simulink model "test_VisionModel_v1"  (Simulink 7.6)
settings: Solver=FixedStepDiscrete  StartTime=0.0  StopTime=0  RelTol=1e-3
values from neighbouring files (symbols this model uses):
  Scale_Down_B = 1    [VisionConstants.m]
  Scale_Down_G = 1    [VisionConstants.m]
  Scale_Down_H = 1    [VisionConstants.m]
  Scale_Down_R = 1    [VisionConstants.m]
  Scale_Down_S = 1    [VisionConstants.m]
  Scale_Down_V = 5    [VisionConstants.m]
  Scale_Forward_B = 0    [VisionConstants.m]
  Scale_Forward_G = 1    [VisionConstants.m]
  Scale_Forward_H = 1    [VisionConstants.m]
  Scale_Forward_R = 0    [VisionConstants.m]
  Scale_Forward_S = 1    [VisionConstants.m]
  Scale_Forward_V = 5    [VisionConstants.m]
undefined symbols (not defined in the file or in its folder): gray, Rec, SDTV
libraries: vipconversions x7, vipsnks x6, vipsrcs x2, viptextngfix x1
settings Model: Creator=Thing 1  LastModifiedBy=auvt
settings OptimizationCC: InlineParams=on  OptimizeModelRefInitCode=on
settings RTWCC: SystemTargetFile=ert.tlc  GenCodeOnly=on  TemplateMakefile=ert_default_tmf  Description=Real-Time Workshop Embedded Coder  GenerateReport=on  ProcessScript=ert_make_rtw_hook  IncludeHyperlinkInReport=on  LaunchReport=on  TargetLang=C++
settings CodeAppCC: IgnoreCustomStorageClasses=off
settings ERTTargetCC: MultiwordLength=2048  GenerateSampleERTMain=on  IncludeMdlTerminateFcn=off  ERTCustomFileTemplate=example_file_process.tlc  ConvertIfToSwitch=off

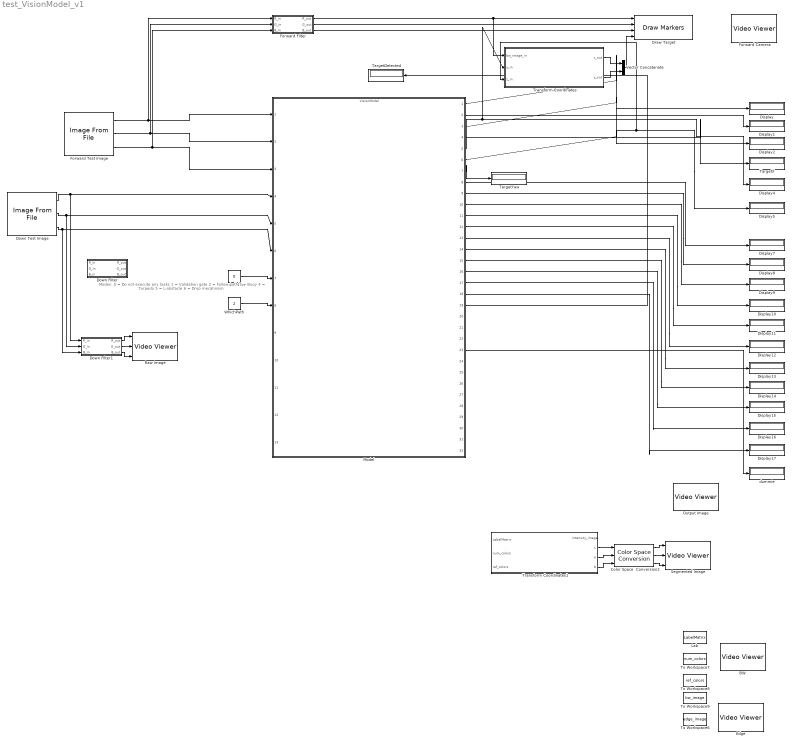
== system test_VisionModel_v1 ==
  note: Modes:
      | 0 = Do not execute any tasks
      | 1 = Validation gate
      | 2 = Follow path
      | 3 = Buoy
      | 4 = Torpedo
      | 5 = L-obstacle
      | 6 = Drop mecahnism
  BW : vipsnks/Video Viewer  DialogControllerArgs=DataTag1  inputType=Obsolete7b  imagePorts=One multidimensional signal  useColorMap=off  colormapValue=gray(256)  specRange=off  minInputVal=0  maxInputVal=255  FigPos=[569 648 462 512]  AxisZoom=on  trueSizedOnce=off  OpenAtMdlStart=on
  Color Space  Conversion2 : vipconversions/Color Space  Conversion  conversion=Obsolete  conversionActive=L*a*b* to sR'G'B'  wp_str=D50  rec=Rec. 601 (SDTV)  sys=1125/60/2:1  imagePorts=Separate color signals
  Display{,1..2,4..5,7..17} (16 alike) : Display
  Down Filter : Subsystem
  Down Filter1 : Subsystem
  Down Test Image : vipsrcs/Image From File  Tag=vipblks_nd  DialogController=vipDDGCreate  DialogControllerArgs=DataTag2  SystemSampleTime=-1  FileName=/home/auvt/auvc/src/vision/Test_Images/path10.bmp  imagePorts=Separate color signals  Ts=-1  ImageDataType=double  Signed=on  WordLength=16  sdImageDataType=uint(8)  FractionLengthMode=User-defined  FractionLength=15  OutPortLabels=R|G|B
  Draw Target : viptextngfix/Draw Markers  DialogController=vipDDGCreate  DialogControllerArgs=DataTag3  shape=X-mark  size=7  fill=off  fillClrSource=Specify via dialog  display=User-specified value  intensity=200  color=[0 0 0]  opacity=0.6  viewport=Entire image  antialiasing=off  inType=Obsolete  imagePorts=Separate color signals  prodOutputMode=Binary point scaling  prodOutputWordLength=32  prodOutputFracLength=14  memoryMode=Specify word length  memoryWordLength=16  memoryFracLength=15  roundingMode=Floor  overflowMode=off
  Edge : vipsnks/Video Viewer  DialogControllerArgs=DataTag5  inputType=Obsolete7b  imagePorts=One multidimensional signal  useColorMap=off  colormapValue=gray(256)  specRange=off  minInputVal=0  maxInputVal=255  FigPos=[58 764 334 594]  AxisZoom=on  trueSizedOnce=off  OpenAtMdlStart=on
  Forward Camera : vipsnks/Video Viewer  DialogControllerArgs=DataTag7  inputType=Obsolete7b  imagePorts=Separate color signals  useColorMap=off  colormapValue=gray(256)  specRange=off  minInputVal=0  maxInputVal=255  FigPos=[1018 735 364 553]  AxisZoom=on  trueSizedOnce=off  OpenAtMdlStart=on
  Forward Filter : Subsystem
  Forward Test Image : vipsrcs/Image From File  Tag=vipblks_nd  DialogController=vipDDGCreate  DialogControllerArgs=DataTag8  SystemSampleTime=-1  FileName=/home/auvt/auvc/src/vision/Test_Images/gate13.bmp  imagePorts=Separate color signals  Ts=-1  ImageDataType=double  Signed=on  WordLength=16  sdImageDataType=uint(8)  FractionLengthMode=User-defined  FractionLength=15  OutPortLabels=R|G|B
  Lab : ToWorkspace  VariableName=LabelMatrix  SampleTime=-1  SaveFormat=Array
  ModeSelect : Constant  Value=0  SampleTime=-1
  Model : ModelReference  ModelNameDialog=VisionModel  SimulationMode=Accelerator  ModelReferenceVersion=1.469  CopyOfModelName=VisionModel
  Output Image : vipsnks/Video Viewer  DialogControllerArgs=DataTag10  inputType=Obsolete7b  imagePorts=Separate color signals  useColorMap=off  colormapValue=gray(256)  specRange=off  minInputVal=0  maxInputVal=255  FigPos=[957 861 423 448]  AxisZoom=on  trueSizedOnce=off  OpenAtMdlStart=on
  Raw Image : vipsnks/Video Viewer  DialogControllerArgs=DataTag12  inputType=Obsolete7b  imagePorts=Separate color signals  useColorMap=off  colormapValue=gray(256)  specRange=off  minInputVal=0  maxInputVal=255  FigPos=[110 703 515 461]  AxisZoom=on  trueSizedOnce=off  OpenAtMdlStart=on
  Segmented Image : vipsnks/Video Viewer  DialogControllerArgs=DataTag14  inputType=Obsolete7b  imagePorts=Separate color signals  useColorMap=off  colormapValue=gray(256)  specRange=off  minInputVal=0  maxInputVal=255  FigPos=[955 778 266 280]  AxisZoom=on  trueSizedOnce=off  OpenAtMdlStart=on
  TargetDetected : Display
  TargetX : Display
  TargetYaw : Display
  To Workspace6 : ToWorkspace  VariableName=edge_image  SampleTime=-1  SaveFormat=Array
  To Workspace7 : ToWorkspace  VariableName=num_colors  SampleTime=-1  SaveFormat=Array
  To Workspace8 : ToWorkspace  VariableName=ref_colors  SampleTime=-1  SaveFormat=Array
  To Workspace9 : ToWorkspace  VariableName=bw_image  SampleTime=-1  SaveFormat=Array
  Transform Coordinates : Stateflow chart  TreatAsAtomicUnit=on  SystemSampleTime=[1/30 0]
  Transform Coordinates1 : Stateflow chart  TreatAsAtomicUnit=on  SystemSampleTime=[1/30 0]
  Vector Concatenate : Concatenate  Mode=Multidimensional array
  WhichPath : Constant  Value=2  SampleTime=-1
  dummie : Display
  wires:
  Down Test Image/1 -> Model/4, Down Filter1/1(R_in)
  Down Test Image/2 -> Model/5, Down Filter1/2(G_in)
  Down Test Image/3 -> Model/6, Down Filter1/3(B_in)
  Model/1 -> Display/1
  Model/2 -> Display1/1
  Model/3 -> Display2/1
  Model/4 -> TargetX/1
  Model/8 -> Display7/1
  Model/9 -> Display8/1
  Model/10 -> Display9/1
  Model/11 -> Display10/1
  Model/12 -> Display11/1
  Model/13 -> Display12/1
  Model/14 -> Display13/1
  Model/15 -> Display14/1
  Model/16 -> Display15/1
  Model/17 -> Display16/1
  Model/18 -> Display17/1
  Transform Coordinates/1(x_out) -> Vector Concatenate/1
  Transform Coordinates/2(y_out) -> Vector Concatenate/2
  Vector Concatenate/1 -> Draw Target/4
  Forward Filter/1(R_out) -> Draw Target/1, Transform Coordinates/1(bw_image_in)
  Forward Filter/2(G_out) -> Draw Target/2
  Forward Filter/3(B_out) -> Draw Target/3
  Model/19 -> TargetDetected/1
  Model/23 -> dummie/1
  Model/5 -> Display4/1, Transform Coordinates/2(y_in)
  Model/6 -> Display5/1, Transform Coordinates/3(z_in)
  Forward Test Image/1 -> Model/1, Forward Filter/1(R_in)
  Forward Test Image/2 -> Model/2, Forward Filter/2(G_in)
  Forward Test Image/3 -> Model/3, Forward Filter/3(B_in)
  ModeSelect/1 -> Model/7
  WhichPath/1 -> Model/8
  Color Space  Conversion2/1 -> Segmented Image/1
  Color Space  Conversion2/2 -> Segmented Image/2
  Color Space  Conversion2/3 -> Segmented Image/3
  Transform Coordinates1/2(L) -> Color Space  Conversion2/1
  Transform Coordinates1/3(a) -> Color Space  Conversion2/2
  Transform Coordinates1/4(b) -> Color Space  Conversion2/3
  Model/7 -> TargetYaw/1
  Down Filter1/2(G_out) -> Raw Image/2
  Down Filter1/1(R_out) -> Raw Image/1
  Down Filter1/3(B_out) -> Raw Image/3

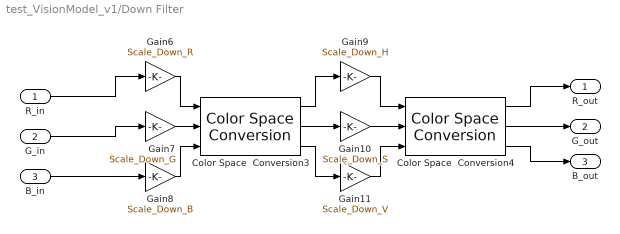
== system test_VisionModel_v1/Down Filter ==
  R_in : Inport  PortDimensions=Down_Camera_Dimensions
  G_in : Inport  Port=2  PortDimensions=Down_Camera_Dimensions
  B_in : Inport  Port=3  PortDimensions=Down_Camera_Dimensions
  Color Space  Conversion3 : vipconversions/Color Space  Conversion  conversion=Obsolete  conversionActive=R'G'B' to HSV  wp_str=D50  rec=Rec. 601 (SDTV)  sys=1125/60/2:1  imagePorts=Separate color signals
  Color Space  Conversion4 : vipconversions/Color Space  Conversion  conversion=Obsolete  conversionActive=HSV to R'G'B'  wp_str=D50  rec=Rec. 601 (SDTV)  sys=1125/60/2:1  imagePorts=Separate color signals
  Gain10 : Gain  Gain=Scale_Down_S
  Gain11 : Gain  Gain=Scale_Down_V
  Gain6 : Gain  Gain=Scale_Down_R
  Gain7 : Gain  Gain=Scale_Down_G
  Gain8 : Gain  Gain=Scale_Down_B
  Gain9 : Gain  Gain=Scale_Down_H
  R_out : Outport  OutDataTypeStr=double
  G_out : Outport  Port=2  OutDataTypeStr=double
  B_out : Outport  Port=3  OutDataTypeStr=double
  wires:
  Gain6/1 -> Color Space  Conversion3/1
  Gain7/1 -> Color Space  Conversion3/2
  Gain8/1 -> Color Space  Conversion3/3
  Color Space  Conversion3/1 -> Gain9/1
  Color Space  Conversion3/2 -> Gain10/1
  Color Space  Conversion3/3 -> Gain11/1
  Gain9/1 -> Color Space  Conversion4/1
  Gain10/1 -> Color Space  Conversion4/2
  Gain11/1 -> Color Space  Conversion4/3
  R_in/1 -> Gain6/1
  G_in/1 -> Gain7/1
  B_in/1 -> Gain8/1
  Color Space  Conversion4/1 -> R_out/1
  Color Space  Conversion4/2 -> G_out/1
  Color Space  Conversion4/3 -> B_out/1

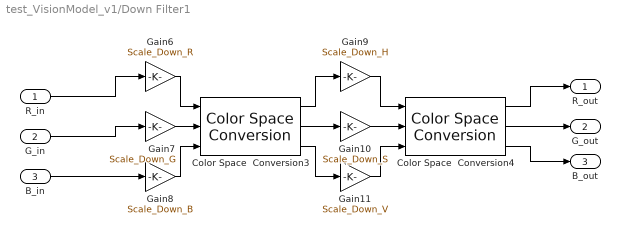
== system test_VisionModel_v1/Down Filter1 ==
  R_in : Inport  PortDimensions=Down_Camera_Dimensions
  G_in : Inport  Port=2  PortDimensions=Down_Camera_Dimensions
  B_in : Inport  Port=3  PortDimensions=Down_Camera_Dimensions
  Color Space  Conversion3 : vipconversions/Color Space  Conversion  conversion=Obsolete  conversionActive=R'G'B' to HSV  wp_str=D50  rec=Rec. 601 (SDTV)  sys=1125/60/2:1  imagePorts=Separate color signals
  Color Space  Conversion4 : vipconversions/Color Space  Conversion  conversion=Obsolete  conversionActive=HSV to R'G'B'  wp_str=D50  rec=Rec. 601 (SDTV)  sys=1125/60/2:1  imagePorts=Separate color signals
  Gain10 : Gain  Gain=Scale_Down_S
  Gain11 : Gain  Gain=Scale_Down_V
  Gain6 : Gain  Gain=Scale_Down_R
  Gain7 : Gain  Gain=Scale_Down_G
  Gain8 : Gain  Gain=Scale_Down_B
  Gain9 : Gain  Gain=Scale_Down_H
  R_out : Outport  OutDataTypeStr=double
  G_out : Outport  Port=2  OutDataTypeStr=double
  B_out : Outport  Port=3  OutDataTypeStr=double
  wires:
  Gain6/1 -> Color Space  Conversion3/1
  Gain7/1 -> Color Space  Conversion3/2
  Gain8/1 -> Color Space  Conversion3/3
  Color Space  Conversion3/1 -> Gain9/1
  Color Space  Conversion3/2 -> Gain10/1
  Color Space  Conversion3/3 -> Gain11/1
  Gain9/1 -> Color Space  Conversion4/1
  Gain10/1 -> Color Space  Conversion4/2
  Gain11/1 -> Color Space  Conversion4/3
  R_in/1 -> Gain6/1
  G_in/1 -> Gain7/1
  B_in/1 -> Gain8/1
  Color Space  Conversion4/1 -> R_out/1
  Color Space  Conversion4/2 -> G_out/1
  Color Space  Conversion4/3 -> B_out/1

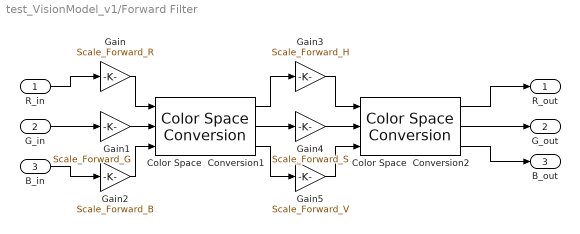
== system test_VisionModel_v1/Forward Filter ==
  R_in : Inport  PortDimensions=Forward_Camera_Dimensions
  G_in : Inport  Port=2  PortDimensions=Forward_Camera_Dimensions
  B_in : Inport  Port=3  PortDimensions=Forward_Camera_Dimensions
  Color Space  Conversion1 : vipconversions/Color Space  Conversion  conversion=Obsolete  conversionActive=R'G'B' to HSV  wp_str=D50  rec=Rec. 601 (SDTV)  sys=1125/60/2:1  imagePorts=Separate color signals
  Color Space  Conversion2 : vipconversions/Color Space  Conversion  conversion=Obsolete  conversionActive=HSV to R'G'B'  wp_str=D50  rec=Rec. 601 (SDTV)  sys=1125/60/2:1  imagePorts=Separate color signals
  Gain : Gain  Gain=Scale_Forward_R
  Gain1 : Gain  Gain=Scale_Forward_G
  Gain2 : Gain  Gain=Scale_Forward_B
  Gain3 : Gain  Gain=Scale_Forward_H
  Gain4 : Gain  Gain=Scale_Forward_S
  Gain5 : Gain  Gain=Scale_Forward_V
  R_out : Outport  OutDataTypeStr=double
  G_out : Outport  Port=2  OutDataTypeStr=double
  B_out : Outport  Port=3  OutDataTypeStr=double
  wires:
  R_in/1 -> Gain/1
  G_in/1 -> Gain1/1
  B_in/1 -> Gain2/1
  Gain/1 -> Color Space  Conversion1/1
  Gain1/1 -> Color Space  Conversion1/2
  Gain2/1 -> Color Space  Conversion1/3
  Color Space  Conversion1/1 -> Gain3/1
  Color Space  Conversion1/2 -> Gain4/1
  Color Space  Conversion1/3 -> Gain5/1
  Gain3/1 -> Color Space  Conversion2/1
  Gain4/1 -> Color Space  Conversion2/2
  Gain5/1 -> Color Space  Conversion2/3
  Color Space  Conversion2/1 -> R_out/1
  Color Space  Conversion2/2 -> G_out/1
  Color Space  Conversion2/3 -> B_out/1

== matlab function Transform Coordinates1 ==
  data: LabelMatrix input double; intensity_image output double; num_colors input double; ref_colors input double; L output double; a output double; b output double
function [intensity_image, L, a, b] = displaySegmentedImage(LabelMatrix, num_colors, ref_colors)


intensity_image = LabelMatrix./max(max(max(abs(LabelMatrix))));


[rows, cols] = size(LabelMatrix);

L = zeros(rows, cols);
a = zeros(rows, cols);
b = zeros(rows, cols);

for r = 1:rows
    for c = 1:cols
        L(r,c) = ref_colors(LabelMatrix(r,c), 1);
        a(r,c) = ref_colors(LabelMatrix(r,c), 2);
        b(r,c) = ref_colors(LabelMatrix(r,c), 3);
    end
end

return

== matlab function Transform Coordinates ==
  data: bw_image_in input double; y_in input double; x_out output double; y_out output double; z_in input double
function [x_out, y_out] = transform_G2L(bw_image_in, y_in, z_in)
% This function, "transform Global to Local coordinates," simply transforms
%   global coordinates that are sent to the controller into local
%   coordinates that can be displayed over images.
%
% 5-29-11

[rows, cols] = size(bw_image_in);
x_out = z_in + floor(rows/2);
y_out = y_in + floor(cols/2);

return
